simulink model "SimCurtoCircuitoComCompensacao"  (R2023b)
settings: Solver=ode45  StartTime=0.0  StopTime=0.1  RelTol=1e-3  EnableMultiTasking=on
values from neighbouring files (symbols this model uses):
  ccc1 = Ccc*d    [CarregaDados1km.m]
  ccc2 = Ccc*d    [CarregaDados1km.m]
  ccc3 = Ccc*d    [CarregaDados1km.m]
  cct1 = Cct*d    [CarregaDados1km.m]
  cct2 = Cct*d    [CarregaDados1km.m]
  cct3 = Cct*d    [CarregaDados1km.m]
  cequa1 = 0    [CarregaDados1km.m]
  cequa2 = 0    [CarregaDados1km.m]
  cequa3 = 0    [CarregaDados1km.m]
  le1 = 1e-10    [CarregaDados1km.m]
  le2 = 1e-10    [CarregaDados1km.m]
  lm1 = (imag(Zm)/(2*pi*f))*d    [CarregaDados1km.m]
  lm2 = (imag(Zm)/(2*pi*f))*d    [CarregaDados1km.m]
  lm3 = (imag(Zm)/(2*pi*f))*d    [CarregaDados1km.m]
  lp1 = (imag(Zp)/(2*pi*f))*d    [CarregaDados1km.m]
  lp2 = (imag(Zp)/(2*pi*f))*d    [CarregaDados1km.m]
  lp3 = (imag(Zp)/(2*pi*f))*d    [CarregaDados1km.m]
  NRE2 = 1e-12    [CarregaDados1km.m]
  rm1 = real(Zm)*d    [CarregaDados1km.m]
  rm2 = real(Zm)*d    [CarregaDados1km.m]
  rm3 = real(Zm)*d    [CarregaDados1km.m]
  rp1 = real(Zp)*d    [CarregaDados1km.m]
  rp2 = real(Zp)*d    [CarregaDados1km.m]
  rp3 = real(Zp)*d    [CarregaDados1km.m]
  rtc1 = 10    [CarregaDados1km.m]
  rtc2 = 10    [CarregaDados1km.m]
undefined symbols (not defined in the file or in its folder): Angle, D11, Delta, le, Magnitude, rti1, rti2
libraries: spsSeriesRLCBranchLib x33, spsThreePhaseVIMeasurementLib x12, spsThreePhaseTransformerTwoWindingsLib x6, spsMutualInductanceLib x3, spsThreePhaseSeriesRLCLoadLib x3, spsThreePhaseSourceLib x1, spspowerguiLib x1
settings Model: Creator=laris  LastModifiedBy=Leonardo Felipe
settings SolverCC: AlgebraicLoopSolver=TrustRegion
settings DataIOCC: LimitDataPoints=on  SaveFormat=Array  ReturnWorkspaceOutputs=off
settings OptimizationCC: ReuseModelBlockBuffer=off  LifeSpan=inf
settings DebuggingCC: UnconnectedInputMsg=warning  UnconnectedOutputMsg=warning  UnconnectedLineMsg=warning  SFUnexpectedBacktrackingDiag=warning  SFNoUnconditionalDefaultTransitionDiag=warning  SFExecutionAtInitializationDiag=none  ArithmeticOperatorsInVariantConditions=warning
settings HardwareCC: ProdBitPerPointer=32  ProdBitPerSizeT=32  ProdBitPerPtrDiffT=32  ProdLargestAtomicFloat=None  ProdIntDivRoundTo=Undefined  ProdEndianess=Unspecified  ProdWordSize=32  ProdHWDeviceType=32-bit Generic
settings ModelReferenceCC: EnableRefExpFcnMdlSchedulingChecks=on  PropagateSignalLabelsOutOfModel=off
settings SFSimCC: SimUseLocalCustomCode=off  CustomCodeUndefinedFunction=UseInterfaceOnly
settings RTWCC: RTWUseLocalCustomCode=off  DLArmComputeVersion=19.05
settings CodeAppCC: StateflowObjectComments=on
settings GRTTargetCC: TargetLangStandard=C89/C90 (ANSI)
settings ConfigComp: CovMetricSettings=dw  CovSaveCumulativeToWorkspaceVar=on  CovSaveSingleToWorkspaceVar=on  CovExternalEMLEnable=off
settings SimscapeCC: SimscapeNormalizeSystem=off

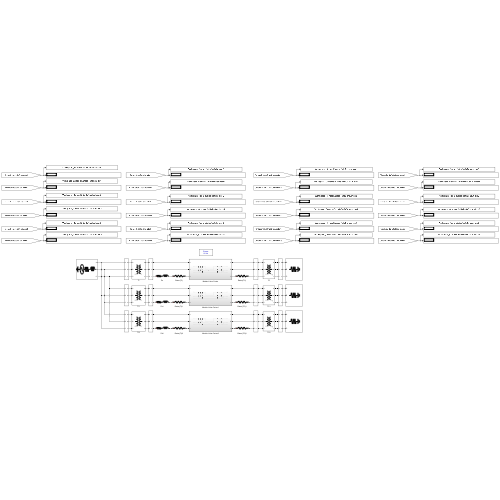
[thumbnail: Simulink's stored preview of the top-level diagram]
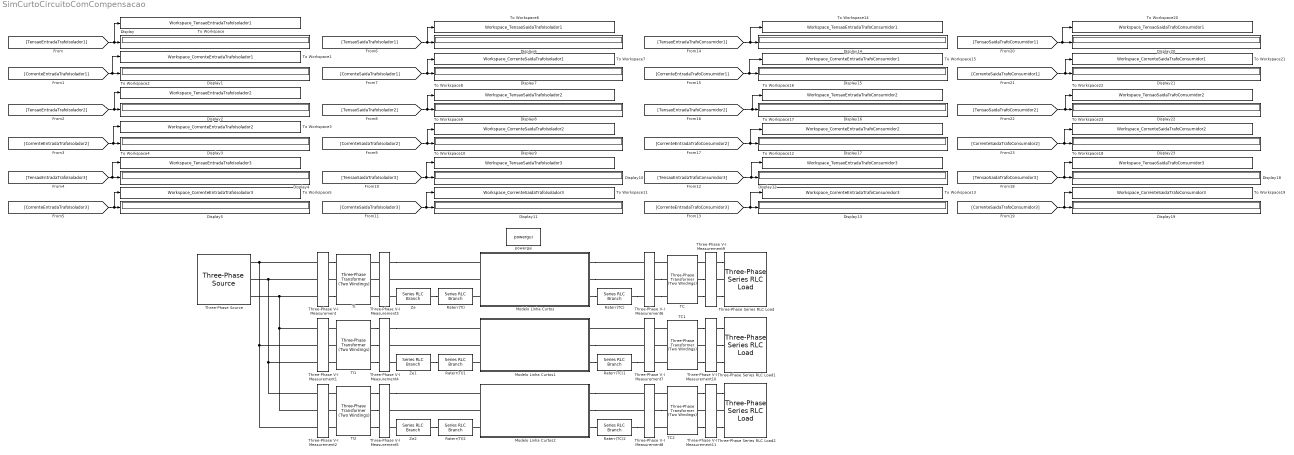
== system SimCurtoCircuitoComCompensacao ==
  Display{,1..23} (24 alike) : Display
  Modelo Linha Curtos : Subsystem
  Modelo Linha Curtos1 : Subsystem
  Modelo Linha Curtos2 : Subsystem
  Raterr(TC) : spsSeriesRLCBranchLib/Series RLC Branch  LConnTagsString=__new0  RConnTagsString=__new0  BranchType=R  Resistance=rtc1  Inductance=0  SetiL0=off  InitialCurrent=0  Capacitance=1e-6  Setx0=off  InitialVoltage=0  Measurements=None
  Raterr(TC)1 : spsSeriesRLCBranchLib/Series RLC Branch  LConnTagsString=__new0  RConnTagsString=__new0  BranchType=R  Resistance=rtc2  Inductance=0  SetiL0=off  InitialCurrent=0  Capacitance=1e-6  Setx0=off  InitialVoltage=0  Measurements=None
  Raterr(TC)2 : spsSeriesRLCBranchLib/Series RLC Branch  LConnTagsString=__new0  RConnTagsString=__new0  BranchType=R  Resistance=rtc2  Inductance=0  SetiL0=off  InitialCurrent=0  Capacitance=1e-6  Setx0=off  InitialVoltage=0  Measurements=None
  Raterr(TI) : spsSeriesRLCBranchLib/Series RLC Branch  LConnTagsString=__new0  RConnTagsString=__new0  BranchType=R  Resistance=rti1  Inductance=0  SetiL0=off  InitialCurrent=0  Capacitance=1e-6  Setx0=off  InitialVoltage=0  Measurements=None
  Raterr(TI)1 : spsSeriesRLCBranchLib/Series RLC Branch  LConnTagsString=__new0  RConnTagsString=__new0  BranchType=R  Resistance=rti2  Inductance=0  SetiL0=off  InitialCurrent=0  Capacitance=1e-6  Setx0=off  InitialVoltage=0  Measurements=None
  Raterr(TI)2 : spsSeriesRLCBranchLib/Series RLC Branch  LConnTagsString=__new0  RConnTagsString=__new0  BranchType=R  Resistance=rti2  Inductance=0  SetiL0=off  InitialCurrent=0  Capacitance=1e-6  Setx0=off  InitialVoltage=0  Measurements=None
  TC : spsThreePhaseTransformerTwoWindingsLib/Three-Phase Transformer (Two Windings)  Winding1Connection=Delta (D11)  Winding2Connection=Yg  CoreType=Three single-phase transformers  SetSaturation=off  Hysteresis=off  DataFile='hysteresis'  SetInitialFlux=off  Measurements=None  UNITS=pu  NominalPower=[120e3 , 60]  Winding1=[13800/sqrt(3) 0.0048118 0.018511]  Winding2=[380 0.0048119 0.018511]  Rm=5.801193266567229e+02*1000  Lm=8.409977380031759e+02*1000  L0=0.50001  Saturation=[0 0;0.0012545 0.01913;0.52272 0.024231]  InitialFluxes=[0.66025 -0.66025 0.57767]  BreakLoop=off  DiscreteSolver=Trapezoidal iterative  DataType=off  TransfoNumber=1
  TC1 : spsThreePhaseTransformerTwoWindingsLib/Three-Phase Transformer (Two Windings)  Winding1Connection=Delta (D11)  Winding2Connection=Yg  CoreType=Three single-phase transformers  SetSaturation=off  Hysteresis=off  DataFile='hysteresis'  SetInitialFlux=off  Measurements=None  UNITS=pu  NominalPower=[120e3 , 60]  Winding1=[13800/sqrt(3) 0.0048118 0.018511]  Winding2=[380 0.0048119 0.018511]  Rm=5.801193266567229e+02*1000  Lm=8.409977380031759e+02*1000  L0=0.50001  Saturation=[0 0;0.0012545 0.01913;0.52272 0.024231]  InitialFluxes=[0.66025 -0.66025 0.57767]  BreakLoop=off  DiscreteSolver=Trapezoidal iterative  DataType=off  TransfoNumber=1
  TC2 : spsThreePhaseTransformerTwoWindingsLib/Three-Phase Transformer (Two Windings)  Winding1Connection=Delta (D11)  Winding2Connection=Yg  CoreType=Three single-phase transformers  SetSaturation=off  Hysteresis=off  DataFile='hysteresis'  SetInitialFlux=off  Measurements=None  UNITS=pu  NominalPower=[120e3 , 60]  Winding1=[13800/sqrt(3) 0.0048118 0.018511]  Winding2=[380 0.0048119 0.018511]  Rm=5.801193266567229e+02*1000  Lm=8.409977380031759e+02*1000  L0=0.50001  Saturation=[0 0;0.0012545 0.01913;0.52272 0.024231]  InitialFluxes=[0.66025 -0.66025 0.57767]  BreakLoop=off  DiscreteSolver=Trapezoidal iterative  DataType=off  TransfoNumber=1
  TI : spsThreePhaseTransformerTwoWindingsLib/Three-Phase Transformer (Two Windings)  Winding1Connection=Delta (D11)  Winding2Connection=Y  CoreType=Three single-phase transformers  SetSaturation=off  Hysteresis=off  DataFile='hysteresis'  SetInitialFlux=off  Measurements=None  UNITS=pu  NominalPower=[300e3 , 60 ]  Winding1=[13800 0.0048119 0.018511]  Winding2=[13800/sqrt(3) 0.0048119 0.018511]  Rm=1.730769230769231e+03*1000  Lm=40.010686750359440*1000  L0=6.3145  Saturation=[0 0;0.0012545 0.01913;0.52272 0.024231]  InitialFluxes=[34.179 -34.179 29.906]  BreakLoop=off  DiscreteSolver=Trapezoidal iterative  DataType=off  TransfoNumber=1
  TI1 : spsThreePhaseTransformerTwoWindingsLib/Three-Phase Transformer (Two Windings)  Winding1Connection=Delta (D11)  Winding2Connection=Y  CoreType=Three single-phase transformers  SetSaturation=off  Hysteresis=off  DataFile='hysteresis'  SetInitialFlux=off  Measurements=None  UNITS=pu  NominalPower=[300e3 , 60 ]  Winding1=[13800 0.0048119 0.018511]  Winding2=[13800/sqrt(3) 0.0048119 0.018511]  Rm=1.730769230769231e+03*1000  Lm=40.010686750359440*1000  L0=6.3145  Saturation=[0 0;0.0012545 0.01913;0.52272 0.024231]  InitialFluxes=[34.179 -34.179 29.906]  BreakLoop=off  DiscreteSolver=Trapezoidal iterative  DataType=off  TransfoNumber=1
  TI2 : spsThreePhaseTransformerTwoWindingsLib/Three-Phase Transformer (Two Windings)  Winding1Connection=Delta (D11)  Winding2Connection=Y  CoreType=Three single-phase transformers  SetSaturation=off  Hysteresis=off  DataFile='hysteresis'  SetInitialFlux=off  Measurements=None  UNITS=pu  NominalPower=[300e3 , 60 ]  Winding1=[13800 0.0048119 0.018511]  Winding2=[13800/sqrt(3) 0.0048119 0.018511]  Rm=1.730769230769231e+03*1000  Lm=40.010686750359440*1000  L0=6.3145  Saturation=[0 0;0.0012545 0.01913;0.52272 0.024231]  InitialFluxes=[34.179 -34.179 29.906]  BreakLoop=off  DiscreteSolver=Trapezoidal iterative  DataType=off  TransfoNumber=1
  Three-Phase Series RLC Load : spsThreePhaseSeriesRLCLoadLib/Three-Phase Series RLC Load  LConnTagsString=A|B|C  Configuration=Y (grounded)  NominalVoltage=220  Vabc=[1e3 1e3 1e3]  Vabcp=[1e3 1e3 1e3]  NominalFrequency=60  UnbalancedPower=off  ActivePower=120e3  InductivePower=0  CapacitivePower=0  Pabc=[10e3 9e3 11e3]  QLabc=[100 90 110]  QCabc=[100 90 110]  Pabcp=[10e3 9e3 11e3]  QLabcp=[100 90 110]  QCabcp=[100 90 110]  Measurements=None  LoadType=constant Z
  Three-Phase Series RLC Load1 : spsThreePhaseSeriesRLCLoadLib/Three-Phase Series RLC Load  LConnTagsString=A|B|C  Configuration=Y (grounded)  NominalVoltage=220  Vabc=[1e3 1e3 1e3]  Vabcp=[1e3 1e3 1e3]  NominalFrequency=60  UnbalancedPower=off  ActivePower=120e3  InductivePower=0  CapacitivePower=0  Pabc=[10e3 9e3 11e3]  QLabc=[100 90 110]  QCabc=[100 90 110]  Pabcp=[10e3 9e3 11e3]  QLabcp=[100 90 110]  QCabcp=[100 90 110]  Measurements=None  LoadType=constant Z
  Three-Phase Series RLC Load2 : spsThreePhaseSeriesRLCLoadLib/Three-Phase Series RLC Load  LConnTagsString=A|B|C  Configuration=Y (grounded)  NominalVoltage=220  Vabc=[1e3 1e3 1e3]  Vabcp=[1e3 1e3 1e3]  NominalFrequency=60  UnbalancedPower=off  ActivePower=120e3  InductivePower=0  CapacitivePower=0  Pabc=[10e3 9e3 11e3]  QLabc=[100 90 110]  QCabc=[100 90 110]  Pabcp=[10e3 9e3 11e3]  QLabcp=[100 90 110]  QCabcp=[100 90 110]  Measurements=None  LoadType=constant Z
  Three-Phase V-I Measurement : spsThreePhaseVIMeasurementLib/Three-Phase V-I Measurement  VoltageMeasurement=phase-to-phase  SetLabelV=on  LabelV=TensaoEntradaTrafoIsolador1  Vpu=off  VpuLL=off  CurrentMeasurement=yes  SetLabelI=on  LabelI=CorrenteEntradaTrafoIsolador1  Ipu=off  Pbase=100e6  Vbase=500e3  OutputType=Magnitude-Angle  PhasorSimulation=on  PSBequivalent=0
  Three-Phase V-I Measurement1 : spsThreePhaseVIMeasurementLib/Three-Phase V-I Measurement  VoltageMeasurement=phase-to-phase  SetLabelV=on  LabelV=TensaoEntradaTrafoIsolador2  Vpu=off  VpuLL=off  CurrentMeasurement=yes  SetLabelI=on  LabelI=CorrenteEntradaTrafoIsolador2  Ipu=off  Pbase=100e6  Vbase=500e3  OutputType=Magnitude-Angle  PhasorSimulation=on  PSBequivalent=0
  Three-Phase V-I Measurement10 : spsThreePhaseVIMeasurementLib/Three-Phase V-I Measurement  VoltageMeasurement=phase-to-phase  SetLabelV=on  LabelV=TensaoSaidaTrafoConsumidor2  Vpu=off  VpuLL=off  CurrentMeasurement=yes  SetLabelI=on  LabelI=CorrenteSaidaTrafoConsumidor2  Ipu=off  Pbase=100e6  Vbase=500e3  OutputType=Magnitude-Angle  PhasorSimulation=on  PSBequivalent=0
  Three-Phase V-I Measurement11 : spsThreePhaseVIMeasurementLib/Three-Phase V-I Measurement  VoltageMeasurement=phase-to-phase  SetLabelV=on  LabelV=TensaoSaidaTrafoConsumidor3  Vpu=off  VpuLL=off  CurrentMeasurement=yes  SetLabelI=on  LabelI=CorrenteSaidaTrafoConsumidor3  Ipu=off  Pbase=100e6  Vbase=500e3  OutputType=Magnitude-Angle  PhasorSimulation=on  PSBequivalent=0
  Three-Phase V-I Measurement2 : spsThreePhaseVIMeasurementLib/Three-Phase V-I Measurement  VoltageMeasurement=phase-to-phase  SetLabelV=on  LabelV=TensaoEntradaTrafoIsolador3  Vpu=off  VpuLL=off  CurrentMeasurement=yes  SetLabelI=on  LabelI=CorrenteEntradaTrafoIsolador3  Ipu=off  Pbase=100e6  Vbase=500e3  OutputType=Magnitude-Angle  PhasorSimulation=on  PSBequivalent=0
  Three-Phase V-I Measurement3 : spsThreePhaseVIMeasurementLib/Three-Phase V-I Measurement  VoltageMeasurement=phase-to-phase  SetLabelV=on  LabelV=TensaoSaidaTrafoIsolador1  Vpu=off  VpuLL=off  CurrentMeasurement=yes  SetLabelI=on  LabelI=CorrenteSaidaTrafoIsolador1  Ipu=off  Pbase=100e6  Vbase=500e3  OutputType=Magnitude-Angle  PhasorSimulation=on  PSBequivalent=0
  Three-Phase V-I Measurement4 : spsThreePhaseVIMeasurementLib/Three-Phase V-I Measurement  VoltageMeasurement=phase-to-phase  SetLabelV=on  LabelV=TensaoSaidaTrafoIsolador2  Vpu=off  VpuLL=off  CurrentMeasurement=yes  SetLabelI=on  LabelI=CorrenteSaidaTrafoIsolador2  Ipu=off  Pbase=100e6  Vbase=500e3  OutputType=Magnitude-Angle  PhasorSimulation=on  PSBequivalent=0
  Three-Phase V-I Measurement5 : spsThreePhaseVIMeasurementLib/Three-Phase V-I Measurement  VoltageMeasurement=phase-to-phase  SetLabelV=on  LabelV=TensaoSaidaTrafoIsolador3  Vpu=off  VpuLL=off  CurrentMeasurement=yes  SetLabelI=on  LabelI=CorrenteSaidaTrafoIsolador3  Ipu=off  Pbase=100e6  Vbase=500e3  OutputType=Magnitude-Angle  PhasorSimulation=on  PSBequivalent=0
  Three-Phase V-I Measurement6 : spsThreePhaseVIMeasurementLib/Three-Phase V-I Measurement  VoltageMeasurement=phase-to-phase  SetLabelV=on  LabelV=TensaoEntradaTrafoConsumidor1  Vpu=off  VpuLL=off  CurrentMeasurement=yes  SetLabelI=on  LabelI=CorrenteEntradaTrafoConsumidor1  Ipu=off  Pbase=100e6  Vbase=500e3  OutputType=Magnitude-Angle  PhasorSimulation=on  PSBequivalent=0
  Three-Phase V-I Measurement7 : spsThreePhaseVIMeasurementLib/Three-Phase V-I Measurement  VoltageMeasurement=phase-to-phase  SetLabelV=on  LabelV=TensaoEntradaTrafoConsumidor2  Vpu=off  VpuLL=off  CurrentMeasurement=yes  SetLabelI=on  LabelI=CorrenteEntradaTrafoConsumidor2  Ipu=off  Pbase=100e6  Vbase=500e3  OutputType=Magnitude-Angle  PhasorSimulation=on  PSBequivalent=0
  Three-Phase V-I Measurement8 : spsThreePhaseVIMeasurementLib/Three-Phase V-I Measurement  VoltageMeasurement=phase-to-phase  SetLabelV=on  LabelV=TensaoEntradaTrafoConsumidor3  Vpu=off  VpuLL=off  CurrentMeasurement=yes  SetLabelI=on  LabelI=CorrenteEntradaTrafoConsumidor3  Ipu=off  Pbase=100e6  Vbase=500e3  OutputType=Magnitude-Angle  PhasorSimulation=on  PSBequivalent=0
  Three-Phase V-I Measurement9 : spsThreePhaseVIMeasurementLib/Three-Phase V-I Measurement  VoltageMeasurement=phase-to-phase  SetLabelV=on  LabelV=TensaoSaidaTrafoConsumidor1  Vpu=off  VpuLL=off  CurrentMeasurement=yes  SetLabelI=on  LabelI=CorrenteSaidaTrafoConsumidor1  Ipu=off  Pbase=100e6  Vbase=500e3  OutputType=Magnitude-Angle  PhasorSimulation=on  PSBequivalent=0
  Three-Phase Source : spsThreePhaseSourceLib/Three-Phase Source  InternalConnection=Yg  VoltagePhases=off  Voltage=13.8e3  PhaseAngle=0  Voltage_phases=[25e3 25e3 25e3]/sqrt(3)  PhaseAngles_phases=[0 -120 +120]  Frequency=60  NonIdealSource=on  SpecifyImpedance=on  Resistance=0.8929  Inductance=16.58e-3  ShortCircuitLevel=120e6  BaseVoltage=13.8e3  XRratio=7  BusType=swing  Pref=10e3  Qref=0  Prefabc=[10e3, 10e3, 10e3]  Qrefabc=[0, 0, 0]  Qmin=-inf  Qmax=inf
  To Workspace : ToWorkspace  VariableName=Workspace_TensaoEntradaTrafoIsolador1  SampleTime=-1
      settings: MaxDataPoints=1
  To Workspace1 : ToWorkspace  VariableName=Workspace_CorrenteEntradaTrafoIsolador1  SampleTime=-1
      settings: MaxDataPoints=1
  To Workspace10 : ToWorkspace  VariableName=Workspace_TensaoSaidaTrafoIsolador3  SampleTime=-1
      settings: MaxDataPoints=1
  To Workspace11 : ToWorkspace  VariableName=Workspace_CorrenteSaidaTrafoIsolador3  SampleTime=-1
      settings: MaxDataPoints=1
  To Workspace12 : ToWorkspace  VariableName=Workspace_TensaoEntradaTrafoConsumidor3  SampleTime=-1
      settings: MaxDataPoints=1
  To Workspace13 : ToWorkspace  VariableName=Workspace_CorrenteEntradaTrafoConsumidor3  SampleTime=-1
      settings: MaxDataPoints=1
  To Workspace14 : ToWorkspace  VariableName=Workspace_TensaoEntradaTrafoConsumidor1  SampleTime=-1
      settings: MaxDataPoints=1
  To Workspace15 : ToWorkspace  VariableName=Workspace_CorrenteEntradaTrafoConsumidor1  SampleTime=-1
      settings: MaxDataPoints=1
  To Workspace16 : ToWorkspace  VariableName=Workspace_TensaoEntradaTrafoConsumidor2  SampleTime=-1
      settings: MaxDataPoints=1
  To Workspace17 : ToWorkspace  VariableName=Workspace_CorrenteEntradaTrafoConsumidor2  SampleTime=-1
      settings: MaxDataPoints=1
  To Workspace18 : ToWorkspace  VariableName=Workspace_TensaoSaidaTrafoConsumidor3  SampleTime=-1
      settings: MaxDataPoints=1
  To Workspace19 : ToWorkspace  VariableName=Workspace_CorrenteSaidaTrafoConsumidor3  SampleTime=-1
      settings: MaxDataPoints=1
  To Workspace2 : ToWorkspace  VariableName=Workspace_TensaoEntradaTrafoIsolador2  SampleTime=-1
      settings: MaxDataPoints=1
  To Workspace20 : ToWorkspace  VariableName=Workspace_TensaoSaidaTrafoConsumidor1  SampleTime=-1
      settings: MaxDataPoints=1
  To Workspace21 : ToWorkspace  VariableName=Workspace_CorrenteSaidaTrafoConsumidor1  SampleTime=-1
      settings: MaxDataPoints=1
  To Workspace22 : ToWorkspace  VariableName=Workspace_TensaoSaidaTrafoConsumidor2  SampleTime=-1
      settings: MaxDataPoints=1
  To Workspace23 : ToWorkspace  VariableName=Workspace_CorrenteSaidaTrafoConsumidor2  SampleTime=-1
      settings: MaxDataPoints=1
  To Workspace3 : ToWorkspace  VariableName=Workspace_CorrenteEntradaTrafoIsolador2  SampleTime=-1
      settings: MaxDataPoints=1
  To Workspace4 : ToWorkspace  VariableName=Workspace_TensaoEntradaTrafoIsolador3  SampleTime=-1
      settings: MaxDataPoints=1
  To Workspace5 : ToWorkspace  VariableName=Workspace_CorrenteEntradaTrafoIsolador3  SampleTime=-1
      settings: MaxDataPoints=1
  To Workspace6 : ToWorkspace  VariableName=Workspace_TensaoSaidaTrafoIsolador1  SampleTime=-1
      settings: MaxDataPoints=1
  To Workspace7 : ToWorkspace  VariableName=Workspace_CorrenteSaidaTrafoIsolador1  SampleTime=-1
      settings: MaxDataPoints=1
  To Workspace8 : ToWorkspace  VariableName=Workspace_TensaoSaidaTrafoIsolador2  SampleTime=-1
      settings: MaxDataPoints=1
  To Workspace9 : ToWorkspace  VariableName=Workspace_CorrenteSaidaTrafoIsolador2  SampleTime=-1
      settings: MaxDataPoints=1
  Ze : spsSeriesRLCBranchLib/Series RLC Branch  LConnTagsString=__new0  RConnTagsString=__new0  BranchType=RL  Resistance=NRE2  Inductance=le1  SetiL0=off  InitialCurrent=0  Capacitance=le  Setx0=off  InitialVoltage=0  Measurements=None
  Ze1 : spsSeriesRLCBranchLib/Series RLC Branch  LConnTagsString=__new0  RConnTagsString=__new0  BranchType=RL  Resistance=NRE2  Inductance=le2  SetiL0=off  InitialCurrent=0  Capacitance=le  Setx0=off  InitialVoltage=0  Measurements=None
  Ze2 : spsSeriesRLCBranchLib/Series RLC Branch  LConnTagsString=__new0  RConnTagsString=__new0  BranchType=RL  Resistance=NRE2  Inductance=le2  SetiL0=off  InitialCurrent=0  Capacitance=le  Setx0=off  InitialVoltage=0  Measurements=None
  powergui : spspowerguiLib/powergui  Priority=1  SimulationMode=Phasor  SampleTime=50e-6  frequency=60  Iterations=50  frequencyindice=60  Pbase=100e6  ErrMax=1e-4  UnitsV=kV  UnitsW=MW  buscounter=0  FunctionMessages=off  echomessages=off  EnableUseOfTLC=off  CurrentSourceSwitches=off  DisableSnubberDevices=off  DisableRonSwitches=off  DisableVfSwitches=off  DisplayEquations=off  AutomaticDiscreteSolvers=off  SolverType=Tustin/Backward Euler (TBE)  Interpol=off  ExternalGateDelay=off  methode=off  Ts=100  x0status=blocks  SPID=on  SwTol=0  HookPort=off  NonlinearTolerance=1e-4  nMaxIteration=100  ContinueOnMaxIteration=off  RestoreLinks=warning  ResistiveCurrentMeasurement=off  Frange=[0:2:500]  Ylog=off  Xlog=on  ShowGrid=off  save=off  variable=ZData  structure=0  ZoomFFT=off  StartTime=0.0  cycles=1  DisplayStyle=1  fundamental=60  FreqAxis=off  MaxFrequency=1000  frequencyindicesteady=1  RmsSteady=1  display=off
  wires:
  [TensaoEntradaTrafoIsolador1] -> To Workspace/1, Display/1
  [CorrenteEntradaTrafoIsolador1] -> To Workspace1/1, Display1/1
  [CorrenteEntradaTrafoIsolador2] -> To Workspace3/1, Display3/1
  [TensaoEntradaTrafoIsolador2] -> To Workspace2/1, Display2/1
  [CorrenteEntradaTrafoIsolador3] -> To Workspace5/1, Display5/1
  [TensaoEntradaTrafoIsolador3] -> To Workspace4/1, Display4/1
  [CorrenteSaidaTrafoIsolador3] -> To Workspace11/1, Display11/1
  [CorrenteSaidaTrafoIsolador1] -> To Workspace7/1, Display7/1
  [TensaoSaidaTrafoIsolador3] -> To Workspace10/1, Display10/1
  [TensaoSaidaTrafoIsolador1] -> To Workspace6/1, Display6/1
  [TensaoSaidaTrafoIsolador2] -> To Workspace8/1, Display8/1
  [CorrenteSaidaTrafoIsolador2] -> To Workspace9/1, Display9/1
  [CorrenteEntradaTrafoConsumidor3] -> To Workspace13/1, Display13/1
  [TensaoEntradaTrafoConsumidor3] -> To Workspace12/1, Display12/1
  [TensaoEntradaTrafoConsumidor2] -> To Workspace16/1, Display16/1
  [CorrenteEntradaTrafoConsumidor2] -> To Workspace17/1, Display17/1
  [CorrenteEntradaTrafoConsumidor1] -> To Workspace15/1, Display15/1
  [TensaoEntradaTrafoConsumidor1] -> To Workspace14/1, Display14/1
  [TensaoSaidaTrafoConsumidor3] -> To Workspace18/1, Display18/1
  [TensaoSaidaTrafoConsumidor1] -> To Workspace20/1, Display20/1
  [TensaoSaidaTrafoConsumidor2] -> To Workspace22/1, Display22/1
  [CorrenteSaidaTrafoConsumidor3] -> To Workspace19/1, Display19/1
  [CorrenteSaidaTrafoConsumidor2] -> To Workspace23/1, Display23/1
  [CorrenteSaidaTrafoConsumidor1] -> To Workspace21/1, Display21/1
  connections:
  Modelo Linha Curtos/RConn1 -- Three-Phase V-I Measurement6/LConn1
  Modelo Linha Curtos/RConn2 -- Three-Phase V-I Measurement6/LConn2
  Raterr(TC)/RConn1 -- Three-Phase V-I Measurement6/LConn3
  Three-Phase V-I Measurement1/LConn1 -- Three-Phase V-I Measurement2/LConn2 -- Three-Phase V-I Measurement/LConn3 -- Three-Phase Source/RConn3
  Three-Phase Source/RConn1 -- Three-Phase V-I Measurement2/LConn3 -- Three-Phase V-I Measurement1/LConn2 -- Three-Phase V-I Measurement/LConn1
  Modelo Linha Curtos/RConn3 -- Raterr(TC)/LConn1
  Three-Phase V-I Measurement/LConn2 -- Three-Phase V-I Measurement2/LConn1 -- Three-Phase V-I Measurement1/LConn3 -- Three-Phase Source/RConn2
  Modelo Linha Curtos/LConn2 -- Three-Phase V-I Measurement3/RConn2
  Ze/RConn1 -- Raterr(TI)/LConn1
  Three-Phase V-I Measurement3/RConn3 -- Ze/LConn1
  Modelo Linha Curtos/LConn3 -- Raterr(TI)/RConn1
  Three-Phase V-I Measurement3/RConn1 -- Modelo Linha Curtos/LConn1
  Three-Phase V-I Measurement4/RConn1 -- Modelo Linha Curtos1/LConn1
  Three-Phase V-I Measurement4/RConn3 -- Ze1/LConn1
  Modelo Linha Curtos1/LConn2 -- Three-Phase V-I Measurement4/RConn2
  Modelo Linha Curtos1/RConn3 -- Raterr(TC)1/LConn1
  Modelo Linha Curtos1/LConn3 -- Raterr(TI)1/RConn1
  Ze1/RConn1 -- Raterr(TI)1/LConn1
  Modelo Linha Curtos2/LConn3 -- Raterr(TI)2/RConn1
  Three-Phase V-I Measurement5/RConn3 -- Ze2/LConn1
  Modelo Linha Curtos2/RConn2 -- Three-Phase V-I Measurement8/LConn2
  Modelo Linha Curtos2/RConn1 -- Three-Phase V-I Measurement8/LConn1
  Ze2/RConn1 -- Raterr(TI)2/LConn1
  Modelo Linha Curtos2/RConn3 -- Raterr(TC)2/LConn1
  Modelo Linha Curtos2/LConn2 -- Three-Phase V-I Measurement5/RConn2
  Three-Phase V-I Measurement5/RConn1 -- Modelo Linha Curtos2/LConn1
  Raterr(TC)2/RConn1 -- Three-Phase V-I Measurement8/LConn3
  Three-Phase V-I Measurement/RConn1 -- TI/LConn1
  TI/LConn2 -- Three-Phase V-I Measurement/RConn2
  Three-Phase V-I Measurement/RConn3 -- TI/LConn3
  TI1/LConn1 -- Three-Phase V-I Measurement1/RConn1
  TI1/LConn3 -- Three-Phase V-I Measurement1/RConn3
  TI1/LConn2 -- Three-Phase V-I Measurement1/RConn2
  TI2/LConn1 -- Three-Phase V-I Measurement2/RConn1
  TI2/LConn2 -- Three-Phase V-I Measurement2/RConn2
  TI2/LConn3 -- Three-Phase V-I Measurement2/RConn3
  Three-Phase V-I Measurement3/LConn1 -- TI/RConn1
  Three-Phase V-I Measurement3/LConn2 -- TI/RConn2
  Three-Phase V-I Measurement3/LConn3 -- TI/RConn3
  TI1/RConn3 -- Three-Phase V-I Measurement4/LConn3
  TI1/RConn1 -- Three-Phase V-I Measurement4/LConn1
  TI1/RConn2 -- Three-Phase V-I Measurement4/LConn2
  TI2/RConn3 -- Three-Phase V-I Measurement5/LConn3
  TI2/RConn2 -- Three-Phase V-I Measurement5/LConn2
  TI2/RConn1 -- Three-Phase V-I Measurement5/LConn1
  TC/LConn1 -- Three-Phase V-I Measurement6/RConn1
  Three-Phase V-I Measurement6/RConn2 -- TC/LConn2
  Three-Phase V-I Measurement6/RConn3 -- TC/LConn3
  Three-Phase V-I Measurement9/LConn1 -- TC/RConn1
  TC/RConn2 -- Three-Phase V-I Measurement9/LConn2
  TC/RConn3 -- Three-Phase V-I Measurement9/LConn3
  Three-Phase V-I Measurement9/RConn1 -- Three-Phase Series RLC Load/LConn1
  Three-Phase Series RLC Load/LConn2 -- Three-Phase V-I Measurement9/RConn2
  Three-Phase V-I Measurement9/RConn3 -- Three-Phase Series RLC Load/LConn3
  Three-Phase V-I Measurement7/LConn1 -- Modelo Linha Curtos1/RConn1
  Modelo Linha Curtos1/RConn2 -- Three-Phase V-I Measurement7/LConn2
  Raterr(TC)1/RConn1 -- Three-Phase V-I Measurement7/LConn3
  TC1/LConn1 -- Three-Phase V-I Measurement7/RConn1
  TC1/LConn2 -- Three-Phase V-I Measurement7/RConn2
  TC1/LConn3 -- Three-Phase V-I Measurement7/RConn3
  Three-Phase V-I Measurement10/LConn2 -- TC1/RConn2
  TC1/RConn1 -- Three-Phase V-I Measurement10/LConn1
  TC1/RConn3 -- Three-Phase V-I Measurement10/LConn3
  Three-Phase V-I Measurement10/RConn1 -- Three-Phase Series RLC Load1/LConn1
  Three-Phase V-I Measurement10/RConn2 -- Three-Phase Series RLC Load1/LConn2
  Three-Phase V-I Measurement10/RConn3 -- Three-Phase Series RLC Load1/LConn3
  TC2/RConn1 -- Three-Phase V-I Measurement11/LConn1
  Three-Phase V-I Measurement11/LConn2 -- TC2/RConn2
  TC2/RConn3 -- Three-Phase V-I Measurement11/LConn3
  Three-Phase V-I Measurement11/RConn1 -- Three-Phase Series RLC Load2/LConn1
  Three-Phase Series RLC Load2/LConn2 -- Three-Phase V-I Measurement11/RConn2
  Three-Phase V-I Measurement11/RConn3 -- Three-Phase Series RLC Load2/LConn3
  TC2/LConn1 -- Three-Phase V-I Measurement8/RConn1
  Three-Phase V-I Measurement8/RConn2 -- TC2/LConn2
  TC2/LConn3 -- Three-Phase V-I Measurement8/RConn3

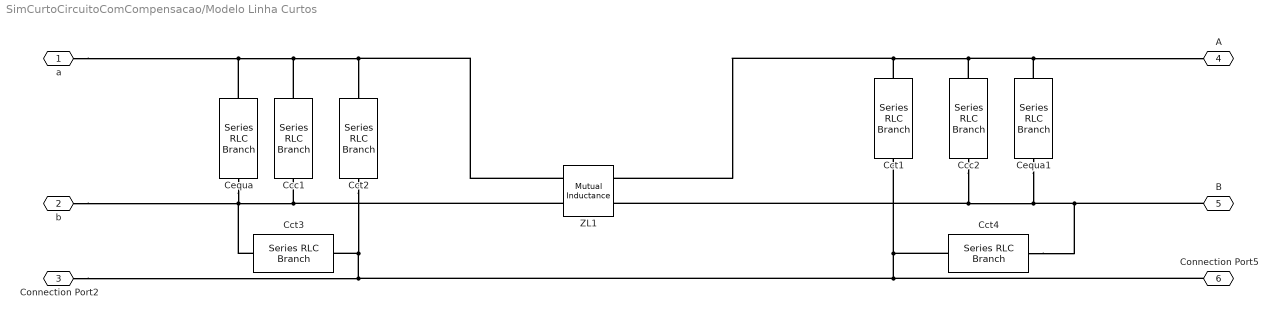
== system SimCurtoCircuitoComCompensacao/Modelo Linha Curtos ==
  Ccc1 : spsSeriesRLCBranchLib/Series RLC Branch  LConnTagsString=__new0  RConnTagsString=__new0  BranchType=C  Resistance=1  Inductance=1e-3  SetiL0=off  InitialCurrent=0  Capacitance=ccc1/2  Setx0=off  InitialVoltage=0  Measurements=Branch voltage
  Ccc2 : spsSeriesRLCBranchLib/Series RLC Branch  LConnTagsString=__new0  RConnTagsString=__new0  BranchType=C  Resistance=1  Inductance=1e-3  SetiL0=off  InitialCurrent=0  Capacitance=ccc1/2  Setx0=off  InitialVoltage=0  Measurements=Branch voltage
  Cct{1..4} (4 alike) : spsSeriesRLCBranchLib/Series RLC Branch  LConnTagsString=__new0  RConnTagsString=__new0  BranchType=C  Resistance=1  Inductance=1e-3  SetiL0=off  InitialCurrent=0  Capacitance=cct1/2  Setx0=off  InitialVoltage=0  Measurements=None
  Cequa : spsSeriesRLCBranchLib/Series RLC Branch  LConnTagsString=__new0  RConnTagsString=__new0  BranchType=C  Resistance=1  Inductance=1e-3  SetiL0=off  InitialCurrent=0  Capacitance=cequa1/2  Setx0=off  InitialVoltage=0  Measurements=None
  Cequa1 : spsSeriesRLCBranchLib/Series RLC Branch  LConnTagsString=__new0  RConnTagsString=__new0  BranchType=C  Resistance=1  Inductance=1e-3  SetiL0=off  InitialCurrent=0  Capacitance=cequa1/2  Setx0=off  InitialVoltage=0  Measurements=None
  ZL1 : spsMutualInductanceLib/Mutual Inductance  LConnTagsString=a|b  RConnTagsString=A|B  TypeOfMutual=Generalized mutual inductance  NumberOfWindings=2  SelfImpedance1=[1.1 1.1e-03]  SelfImpedance2=[ 1.1 1.1e-03]  ThreeWindings=on  SelfImpedance3=[ 1.1 1.1e-03]  MutualImpedance=[1.0 1.0e-03]  InductanceMatrix=[lp1 lm1 ; lm1 lp1]  ResistanceMatrix=[rp1 rm1 ; rm1 rp1]  Measurements=None
  a : PMIOPort  Side=Left
  b : PMIOPort  Port=2  Side=Left
  Connection Port2 : PMIOPort  Port=3  Side=Left
  A : PMIOPort  Port=4  Side=Right
  B : PMIOPort  Port=5  Side=Right
  Connection Port5 : PMIOPort  Port=6  Side=Right
  connections:
  Ccc1/LConn1 -- Cequa/LConn1 -- a/RConn1 -- ZL1/LConn1 -- Cct2/LConn1
  Cct3/LConn1 -- ZL1/LConn2 -- Ccc1/RConn1 -- Cequa/RConn1 -- b/RConn1
  Connection Port5/RConn1 -- Connection Port2/RConn1 -- Cct2/RConn1 -- Cct3/RConn1 -- Cct4/RConn1 -- Cct1/RConn1
  B/RConn1 -- Cct4/LConn1 -- ZL1/RConn2 -- Ccc2/RConn1 -- Cequa1/RConn1
  Cequa1/LConn1 -- ZL1/RConn1 -- Cct1/LConn1 -- Ccc2/LConn1 -- A/RConn1

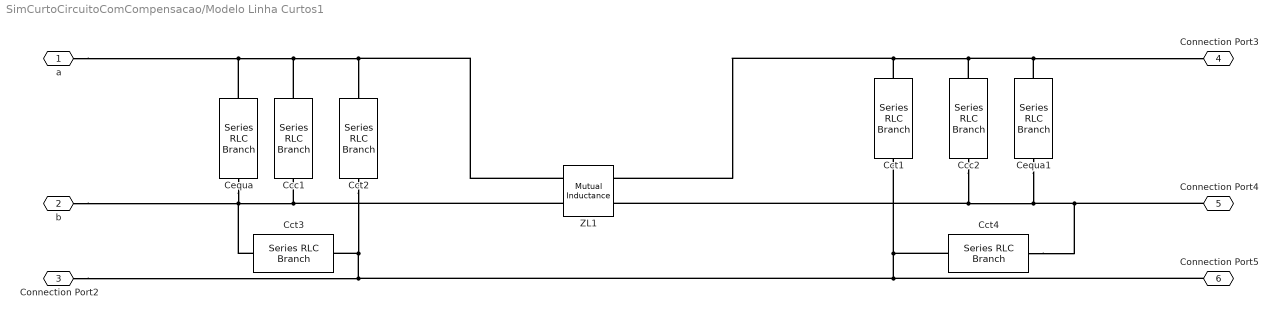
== system SimCurtoCircuitoComCompensacao/Modelo Linha Curtos1 ==
  Ccc1 : spsSeriesRLCBranchLib/Series RLC Branch  LConnTagsString=__new0  RConnTagsString=__new0  BranchType=C  Resistance=1  Inductance=1e-3  SetiL0=off  InitialCurrent=0  Capacitance=ccc2/2  Setx0=off  InitialVoltage=0  Measurements=Branch voltage
  Ccc2 : spsSeriesRLCBranchLib/Series RLC Branch  LConnTagsString=__new0  RConnTagsString=__new0  BranchType=C  Resistance=1  Inductance=1e-3  SetiL0=off  InitialCurrent=0  Capacitance=ccc2/2  Setx0=off  InitialVoltage=0  Measurements=Branch voltage
  Cct{1..4} (4 alike) : spsSeriesRLCBranchLib/Series RLC Branch  LConnTagsString=__new0  RConnTagsString=__new0  BranchType=C  Resistance=1  Inductance=1e-3  SetiL0=off  InitialCurrent=0  Capacitance=cct2/2  Setx0=off  InitialVoltage=0  Measurements=None
  Cequa : spsSeriesRLCBranchLib/Series RLC Branch  LConnTagsString=__new0  RConnTagsString=__new0  BranchType=C  Resistance=1  Inductance=1e-3  SetiL0=off  InitialCurrent=0  Capacitance=cequa2/2  Setx0=off  InitialVoltage=0  Measurements=None
  Cequa1 : spsSeriesRLCBranchLib/Series RLC Branch  LConnTagsString=__new0  RConnTagsString=__new0  BranchType=C  Resistance=1  Inductance=1e-3  SetiL0=off  InitialCurrent=0  Capacitance=cequa2/2  Setx0=off  InitialVoltage=0  Measurements=None
  ZL1 : spsMutualInductanceLib/Mutual Inductance  LConnTagsString=a|b  RConnTagsString=A|B  TypeOfMutual=Generalized mutual inductance  NumberOfWindings=2  SelfImpedance1=[1.1 1.1e-03]  SelfImpedance2=[ 1.1 1.1e-03]  ThreeWindings=on  SelfImpedance3=[ 1.1 1.1e-03]  MutualImpedance=[1.0 1.0e-03]  InductanceMatrix=[lp2 lm2 ; lm2 lp2]  ResistanceMatrix=[rp2 rm2 ; rm2 rp2]  Measurements=None
  a : PMIOPort  Side=Left
  b : PMIOPort  Port=2  Side=Left
  Connection Port2 : PMIOPort  Port=3  Side=Left
  Connection Port3 : PMIOPort  Port=4  Side=Right
  Connection Port4 : PMIOPort  Port=5  Side=Right
  Connection Port5 : PMIOPort  Port=6  Side=Right
  connections:
  Ccc1/LConn1 -- Cequa/LConn1 -- a/RConn1 -- ZL1/LConn1 -- Cct2/LConn1
  Cct3/LConn1 -- ZL1/LConn2 -- Ccc1/RConn1 -- Cequa/RConn1 -- b/RConn1
  Connection Port5/RConn1 -- Connection Port2/RConn1 -- Cct2/RConn1 -- Cct3/RConn1 -- Cct4/RConn1 -- Cct1/RConn1
  Connection Port4/RConn1 -- Cct4/LConn1 -- ZL1/RConn2 -- Ccc2/RConn1 -- Cequa1/RConn1
  Cequa1/LConn1 -- ZL1/RConn1 -- Cct1/LConn1 -- Ccc2/LConn1 -- Connection Port3/RConn1

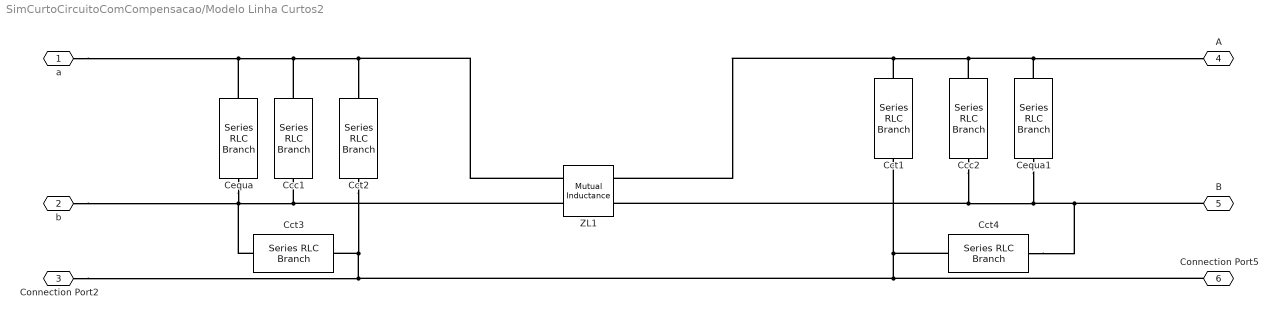
== system SimCurtoCircuitoComCompensacao/Modelo Linha Curtos2 ==
  Ccc1 : spsSeriesRLCBranchLib/Series RLC Branch  LConnTagsString=__new0  RConnTagsString=__new0  BranchType=C  Resistance=1  Inductance=1e-3  SetiL0=off  InitialCurrent=0  Capacitance=ccc3/2  Setx0=off  InitialVoltage=0  Measurements=Branch voltage
  Ccc2 : spsSeriesRLCBranchLib/Series RLC Branch  LConnTagsString=__new0  RConnTagsString=__new0  BranchType=C  Resistance=1  Inductance=1e-3  SetiL0=off  InitialCurrent=0  Capacitance=ccc3/2  Setx0=off  InitialVoltage=0  Measurements=Branch voltage
  Cct{1..4} (4 alike) : spsSeriesRLCBranchLib/Series RLC Branch  LConnTagsString=__new0  RConnTagsString=__new0  BranchType=C  Resistance=1  Inductance=1e-3  SetiL0=off  InitialCurrent=0  Capacitance=cct3/2  Setx0=off  InitialVoltage=0  Measurements=None
  Cequa : spsSeriesRLCBranchLib/Series RLC Branch  LConnTagsString=__new0  RConnTagsString=__new0  BranchType=C  Resistance=1  Inductance=1e-3  SetiL0=off  InitialCurrent=0  Capacitance=cequa3/2  Setx0=off  InitialVoltage=0  Measurements=None
  Cequa1 : spsSeriesRLCBranchLib/Series RLC Branch  LConnTagsString=__new0  RConnTagsString=__new0  BranchType=C  Resistance=1  Inductance=1e-3  SetiL0=off  InitialCurrent=0  Capacitance=cequa3/2  Setx0=off  InitialVoltage=0  Measurements=None
  ZL1 : spsMutualInductanceLib/Mutual Inductance  LConnTagsString=a|b  RConnTagsString=A|B  TypeOfMutual=Generalized mutual inductance  NumberOfWindings=2  SelfImpedance1=[1.1 1.1e-03]  SelfImpedance2=[ 1.1 1.1e-03]  ThreeWindings=on  SelfImpedance3=[ 1.1 1.1e-03]  MutualImpedance=[1.0 1.0e-03]  InductanceMatrix=[lp3 lm3 ; lm3 lp3]  ResistanceMatrix=[rp3 rm3 ; rm3 rp3]  Measurements=None
  a : PMIOPort  Side=Left
  b : PMIOPort  Port=2  Side=Left
  Connection Port2 : PMIOPort  Port=3  Side=Left
  A : PMIOPort  Port=4  Side=Right
  B : PMIOPort  Port=5  Side=Right
  Connection Port5 : PMIOPort  Port=6  Side=Right
  connections:
  Ccc1/LConn1 -- Cequa/LConn1 -- a/RConn1 -- ZL1/LConn1 -- Cct2/LConn1
  Cct3/LConn1 -- ZL1/LConn2 -- Ccc1/RConn1 -- Cequa/RConn1 -- b/RConn1
  Connection Port5/RConn1 -- Connection Port2/RConn1 -- Cct2/RConn1 -- Cct3/RConn1 -- Cct4/RConn1 -- Cct1/RConn1
  B/RConn1 -- Cct4/LConn1 -- ZL1/RConn2 -- Ccc2/RConn1 -- Cequa1/RConn1
  Cequa1/LConn1 -- ZL1/RConn1 -- Cct1/LConn1 -- Ccc2/LConn1 -- A/RConn1
